simulink model "sampleModel1600"  (R2023a)
settings: Solver=VariableStepAuto  StartTime=0.0  StopTime=10.0  RelTol=1e-3
libraries: hdlsllib x2, simulink x1
settings Model: Creator=user1  LastModifiedBy=user1

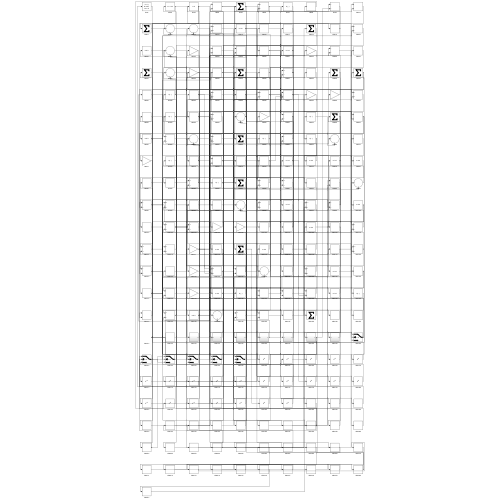
[thumbnail: Simulink's stored preview of the top-level diagram]
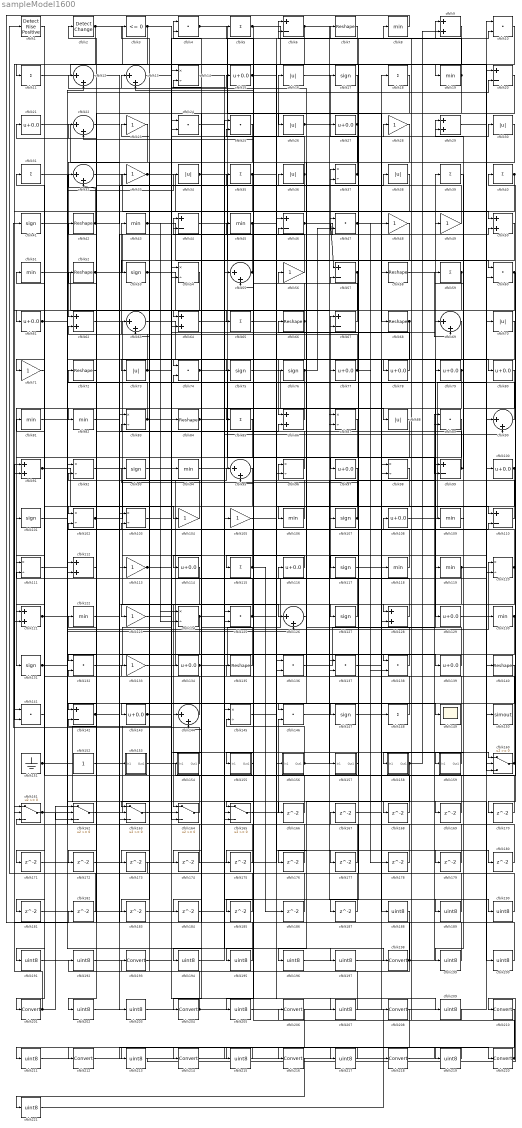
== system sampleModel1600 ==
  cfblk1 : hdlsllib/Logic and Bit Operations/Detect Rise Positive  vinit=0  OutDataTypeStr=boolean
  cfblk{4,10,24..25,47,60,74,89,125,132,136..138,141,146} (15 alike) : DotProduct  OutDataTypeStr=Inherit: Inherit via internal rule
  cfblk{15,21,27,61,77..80,97,100,108,114,116,129,134,139,143} (17 alike) : Bias  Bias=0.0  SaturateOnIntegerOverflow=off
  cfblk{17,41,53,75..76,93,101,107,117,127,131,147} (12 alike) : Signum
  cfblk{14,37,54,83,87,92,96,98,102..103,111,120,124,145} (14 alike) : Product  Inputs=*/  RndMeth=Zero  SaturateOnIntegerOverflow=on
  cfblk{23,28,33,48..49,56,71,104..105,113,123,133} (12 alike) : Gain
  cfblk{8,19,43,45,51,81..82,94,106,109,118..119,122,130} (14 alike) : MinMax
  cfblk{5,11,18,31,35,39..40,59,65,85,115,148} (12 alike) : Sum  Inputs=+
  cfblk{6,20,44,46,57,67,99,110,142} (9 alike) : Sum  Inputs=+-
  cfblk{9,29,50,62,64,86,91,112,121,128} (10 alike) : Sum
  cfblk{12..13,22,32,55,63,69,90,95,126,144} (11 alike) : Sum  Inputs=|++
  cfblk{7,42,52,58,66,68,72,84,135,140} (10 alike) : Reshape
  cfblk149 : Scope
  cfblk150 : ToWorkspace  VariableName=simout  SaveFormat=Timeseries  SampleTime=-1
  cfblk151 : Ground
  cfblk152 : Constant  SampleTime=-1
  cfblk153 : Subsystem
      settings: LibrarySourceBlock=|
      | hdlsllib/Ports &
      | Subsystems/Subsystem
  cfblk154 : Subsystem
      settings: LibrarySourceBlock=|
      | hdlsllib/Ports &
      | Subsystems/Subsystem
  cfblk155 : Subsystem
      settings: LibrarySourceBlock=|
      | hdlsllib/Ports &
      | Subsystems/Subsystem
  cfblk156 : Subsystem
      settings: LibrarySourceBlock=|
      | hdlsllib/Ports &
      | Subsystems/Subsystem
  cfblk157 : Subsystem
      settings: LibrarySourceBlock=|
      | hdlsllib/Ports &
      | Subsystems/Subsystem
  cfblk158 : Subsystem
      settings: LibrarySourceBlock=|
      | hdlsllib/Ports &
      | Subsystems/Subsystem
  cfblk159 : Subsystem
      settings: LibrarySourceBlock=|
      | hdlsllib/Ports &
      | Subsystems/Subsystem
  cfblk{16,26,30,34,36,38,70,73,88} (9 alike) : Abs  SaturateOnIntegerOverflow=off
  cfblk{160..165} (6 alike) : Switch  SaturateOnIntegerOverflow=off  InputSameDT=off
  cfblk{166..187} (22 alike) : Delay  SampleTime=1
  cfblk{188..192,194..197,199..200,202..203,205,207,209,211,213,215,217,219,221} (22 alike) : DataTypeConversion  OutDataTypeStr=uint8  SaturateOnIntegerOverflow=off  RndMeth=Floor
  cfblk{193,198,201,204,206,208,210,212,214,216,218,220} (12 alike) : DataTypeConversion  SaturateOnIntegerOverflow=off  RndMeth=Floor
  cfblk2 : simulink/Logic and Bit Operations/Detect Change  vinit=0  OutDataTypeStr=boolean
      settings: LibrarySourceBlock=|
      | hdlsllib/Logic and Bit
      | Operations/Detect
      | Change
  cfblk3 : hdlsllib/Logic and Bit Operations/Compare To Zero  relop=<=  OutDataTypeStr=boolean
  wires:
  cfblk125/1 -> cfblk123/1, cfblk37/2, cfblk103/2
  cfblk23/1 -> cfblk62/1
  cfblk76/1 -> cfblk131/1, cfblk47/2
  cfblk128/1 -> cfblk67/1
  cfblk30/1 -> cfblk64/1
  cfblk73/1 -> cfblk43/1, cfblk138/1
  cfblk136/1 -> cfblk39/1
  cfblk70/1 -> cfblk78/1
  cfblk106/1 -> cfblk44/1
  cfblk94/1 -> cfblk6/1
  cfblk154/1(Out1) -> cfblk41/1
  cfblk153/1(Out1) -> cfblk40/1
  cfblk13/1 -> cfblk94/1
  cfblk3/1 -> cfblk11/1, cfblk75/1, cfblk121/1
  cfblk115/1 -> cfblk23/1, cfblk186/1
  cfblk92/1 -> cfblk164/1
  cfblk80/1 -> cfblk158/1(In1)
  cfblk133/1 -> cfblk95/1
  cfblk120/1 -> cfblk108/1, cfblk165/3
  cfblk132/1 -> cfblk84/1
  cfblk6/1 -> cfblk71/1, cfblk180/1
  cfblk17/1 -> cfblk132/1
  cfblk27/1 -> cfblk106/1, cfblk26/1
  cfblk57/1 -> cfblk74/1, cfblk165/2
  cfblk62/1 -> cfblk104/1
  cfblk20/1 -> cfblk97/1
  cfblk103/1 -> cfblk28/1
  cfblk99/1 -> cfblk32/1, cfblk59/1
  cfblk104/1 -> cfblk42/1
  cfblk163/1 -> cfblk116/1
  cfblk110/1 -> cfblk67/2
  cfblk129/1 -> cfblk120/1
  cfblk107/1 -> cfblk93/1, cfblk13/2
  cfblk142/1 -> cfblk2/1, cfblk86/2
  cfblk131/1 -> cfblk130/1, cfblk126/2, cfblk163/3
  cfblk37/1 -> cfblk17/1, cfblk187/1
  cfblk98/1 -> cfblk201/1
  cfblk63/1 -> cfblk129/1
  cfblk32/1 -> cfblk50/1
  cfblk139/1 -> cfblk33/1
  cfblk114/1 -> cfblk144/1
  cfblk148/1 -> cfblk63/1
  cfblk74/1 -> cfblk118/1, cfblk136/2
  cfblk95/1 -> cfblk114/1
  cfblk44/1 -> cfblk16/1
  cfblk140/1 -> cfblk143/1
  cfblk69/1 -> cfblk86/1
  cfblk97/1 -> cfblk146/1
  cfblk160/1 -> cfblk56/1, cfblk83/2
  cfblk156/1(Out1) -> cfblk25/2, cfblk99/1
  cfblk42/1 -> cfblk32/2, cfblk36/1
  cfblk83/1 -> cfblk69/1, cfblk72/1
  cfblk26/1 -> cfblk87/1, cfblk99/2
  cfblk51/1 -> cfblk125/1
  cfblk88/1 -> cfblk101/1
  cfblk124/1 -> cfblk134/1, cfblk160/3
  cfblk164/1 -> cfblk81/1
  cfblk40/1 -> cfblk111/1, cfblk205/1
  cfblk54/1 -> cfblk102/1
  cfblk77/1 -> cfblk62/2, cfblk138/2
  cfblk147/1 -> cfblk48/1
  cfblk41/1 -> cfblk139/1
  cfblk79/1 -> cfblk29/1, cfblk112/2
  cfblk100/1 -> cfblk127/1, cfblk184/1
  cfblk4/1 -> cfblk68/1, cfblk156/1(In1)
  cfblk87/1 -> cfblk162/2
  cfblk35/1 -> cfblk82/1, cfblk91/2, cfblk179/1
  cfblk61/1 -> cfblk34/1, cfblk168/1
  cfblk90/1 -> cfblk13/1
  cfblk9/1 -> cfblk64/2
  cfblk113/1 -> cfblk27/1, cfblk124/2, cfblk29/2
  cfblk11/1 -> cfblk19/1
  cfblk138/1 -> cfblk12/1
  cfblk86/1 -> cfblk85/1
  cfblk60/1 -> cfblk159/1(In1), cfblk121/2, cfblk170/1
  cfblk64/1 -> cfblk49/1
  cfblk112/1 -> cfblk52/1
  cfblk53/1 -> cfblk157/1(In1), cfblk147/1
  cfblk78/1 -> cfblk66/1
  cfblk31/1 -> cfblk80/1
  cfblk165/1 -> cfblk146/2
  cfblk38/1 -> cfblk155/1(In1)
  cfblk161/1 -> cfblk79/1, cfblk162/3
  cfblk10/1 -> cfblk117/1
  cfblk52/1 -> cfblk37/1, cfblk137/2
  cfblk18/1 -> cfblk204/1
  cfblk58/1 -> cfblk69/2
  cfblk33/1 -> cfblk140/1, cfblk63/2
  cfblk126/1 -> cfblk96/1
  cfblk65/1 -> cfblk96/2
  cfblk108/1 -> cfblk20/1
  cfblk46/1 -> cfblk57/1, cfblk50/2
  cfblk7/1 -> cfblk61/1
  cfblk144/1 -> cfblk51/1
  cfblk14/1 -> cfblk198/1
  cfblk141/1 -> cfblk31/1
  cfblk101/1 -> cfblk149/1
  cfblk134/1 -> cfblk10/1, cfblk154/1(In1)
  cfblk39/1 -> cfblk109/1
  cfblk22/1 -> cfblk65/1
  cfblk59/1 -> cfblk87/2, cfblk76/1
  cfblk152/1 -> cfblk113/1
  cfblk162/1 -> cfblk30/1
  cfblk16/1 -> cfblk137/1
  cfblk66/1 -> cfblk73/1, cfblk22/2
  cfblk151/1 -> cfblk9/1, cfblk200/1, cfblk203/1
  cfblk12/1 -> cfblk126/1
  cfblk2/1 -> cfblk141/2, cfblk107/1
  cfblk91/1 -> cfblk164/2, cfblk20/2
  cfblk43/1 -> cfblk150/1, cfblk124/1
  cfblk123/1 -> cfblk54/2
  cfblk116/1 -> cfblk115/1
  cfblk28/1 -> cfblk163/1
  cfblk145/1 -> cfblk119/1
  cfblk158/1(Out1) -> cfblk9/2, cfblk176/1, cfblk196/1
  cfblk34/1 -> cfblk60/1, cfblk88/1
  cfblk93/1 -> cfblk77/1
  cfblk122/1 -> cfblk83/1
  cfblk84/1 -> cfblk55/1, cfblk38/1
  cfblk82/1 -> cfblk47/1
  cfblk130/1 -> cfblk164/3, cfblk163/2
  cfblk135/1 -> cfblk4/1
  cfblk118/1 -> cfblk92/2
  cfblk29/1 -> cfblk120/2
  cfblk67/1 -> cfblk45/1
  cfblk111/1 -> cfblk12/2
  cfblk157/1(Out1) -> cfblk7/1
  cfblk45/1 -> cfblk10/2, cfblk173/1
  cfblk143/1 -> cfblk15/1, cfblk160/1
  cfblk47/1 -> cfblk60/2, cfblk178/1
  cfblk56/1 -> cfblk35/1
  cfblk36/1 -> cfblk5/1, cfblk202/1
  cfblk127/1 -> cfblk111/2
  cfblk49/1 -> cfblk21/1
  cfblk119/1 -> cfblk90/1, cfblk128/1
  cfblk15/1 -> cfblk110/1, cfblk177/1
  cfblk96/1 -> cfblk44/2
  cfblk19/1 -> cfblk6/2, cfblk194/1
  cfblk5/1 -> cfblk100/1, cfblk185/1
  cfblk155/1(Out1) -> cfblk135/1
  cfblk21/1 -> cfblk153/1(In1)
  cfblk121/1 -> cfblk110/2, cfblk197/1
  cfblk68/1 -> cfblk128/2, cfblk175/1
  cfblk55/1 -> cfblk165/1, cfblk53/1
  cfblk75/1 -> cfblk148/1
  cfblk117/1 -> cfblk58/1
  cfblk25/1 -> cfblk142/1
  cfblk159/1(Out1) -> cfblk22/1
  cfblk102/1 -> cfblk46/2, cfblk160/2, cfblk90/2
  cfblk81/1 -> cfblk166/1
  cfblk166/1 -> cfblk92/1
  cfblk168/1 -> cfblk144/2
  cfblk137/1 -> cfblk169/1
  cfblk169/1 -> cfblk55/2
  cfblk170/1 -> cfblk57/2
  cfblk85/1 -> cfblk171/1
  cfblk171/1 -> cfblk136/1
  cfblk72/1 -> cfblk172/1
  cfblk172/1 -> cfblk46/1
  cfblk173/1 -> cfblk1/1
  cfblk48/1 -> cfblk174/1
  cfblk174/1 -> cfblk102/2
  cfblk175/1 -> cfblk4/2
  cfblk176/1 -> cfblk161/3
  cfblk177/1 -> cfblk95/2
  cfblk178/1 -> cfblk74/2
  cfblk179/1 -> cfblk112/1
  cfblk180/1 -> cfblk145/1
  cfblk71/1 -> cfblk181/1
  cfblk181/1 -> cfblk54/1
  cfblk8/1 -> cfblk182/1
  cfblk182/1 -> cfblk141/1
  cfblk50/1 -> cfblk183/1
  cfblk183/1 -> cfblk25/1
  cfblk184/1 -> cfblk125/2
  cfblk185/1 -> cfblk142/2
  cfblk186/1 -> cfblk132/2
  cfblk187/1 -> cfblk161/2
  cfblk167/1 -> cfblk188/1
  cfblk146/1 -> cfblk189/1
  cfblk189/1 -> cfblk167/1
  cfblk24/1 -> cfblk190/1
  cfblk190/1 -> cfblk133/1
  cfblk1/1 -> cfblk191/1
  cfblk191/1 -> cfblk24/1
  cfblk188/1 -> cfblk192/1
  cfblk192/1 -> cfblk24/2
  cfblk194/1 -> cfblk105/1
  cfblk89/1 -> cfblk195/1
  cfblk195/1 -> cfblk122/1
  cfblk196/1 -> cfblk89/1
  cfblk197/1 -> cfblk89/2
  cfblk198/1 -> cfblk103/1, cfblk161/1
  cfblk109/1 -> cfblk199/1
  cfblk199/1 -> cfblk14/1
  cfblk200/1 -> cfblk14/2
  cfblk201/1 -> cfblk91/1, cfblk162/1
  cfblk202/1 -> cfblk98/1
  cfblk203/1 -> cfblk98/2
  cfblk204/1 -> cfblk3/1, cfblk70/1
  cfblk205/1 -> cfblk18/1
  cfblk105/1 -> cfblk207/1
  cfblk207/1 -> cfblk193/1
  cfblk193/1 -> cfblk209/1
  cfblk209/1 -> cfblk206/1
  cfblk206/1 -> cfblk211/1
  cfblk211/1 -> cfblk208/1
  cfblk208/1 -> cfblk213/1
  cfblk213/1 -> cfblk210/1
  cfblk210/1 -> cfblk215/1
  cfblk215/1 -> cfblk212/1
  cfblk212/1 -> cfblk217/1
  cfblk217/1 -> cfblk214/1
  cfblk218/1 -> cfblk220/1
  cfblk214/1 -> cfblk219/1
  cfblk219/1 -> cfblk216/1
  cfblk220/1 -> cfblk8/1, cfblk145/2
  cfblk216/1 -> cfblk221/1
  cfblk221/1 -> cfblk218/1

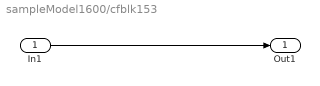
== system sampleModel1600/cfblk153 ==
  In1 : Inport
  Out1 : Outport
  wires:
  In1/1 -> Out1/1

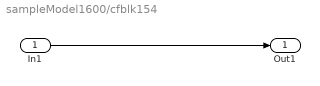
== system sampleModel1600/cfblk154 ==
  In1 : Inport
  Out1 : Outport
  wires:
  In1/1 -> Out1/1

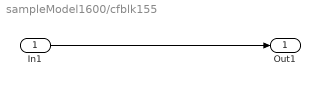
== system sampleModel1600/cfblk155 ==
  In1 : Inport
  Out1 : Outport
  wires:
  In1/1 -> Out1/1

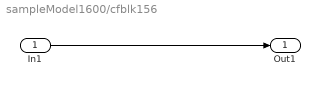
== system sampleModel1600/cfblk156 ==
  In1 : Inport
  Out1 : Outport
  wires:
  In1/1 -> Out1/1

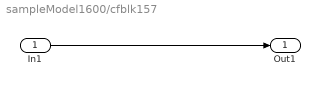
== system sampleModel1600/cfblk157 ==
  In1 : Inport
  Out1 : Outport
  wires:
  In1/1 -> Out1/1

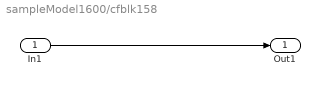
== system sampleModel1600/cfblk158 ==
  In1 : Inport
  Out1 : Outport
  wires:
  In1/1 -> Out1/1

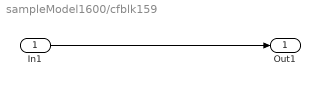
== system sampleModel1600/cfblk159 ==
  In1 : Inport
  Out1 : Outport
  wires:
  In1/1 -> Out1/1
